simulink model "calcul_SA_SR"  (R2024b)
settings: Solver=VariableStepAuto  StartTime=0.0  StopTime=10.0  RelTol=1e-3
values from neighbouring files (symbols this model uses):
  Re = 0.47/2    (= 0.235)    [main_data_vehicle.m]
settings Model: Creator=marti  LastModifiedBy=marti

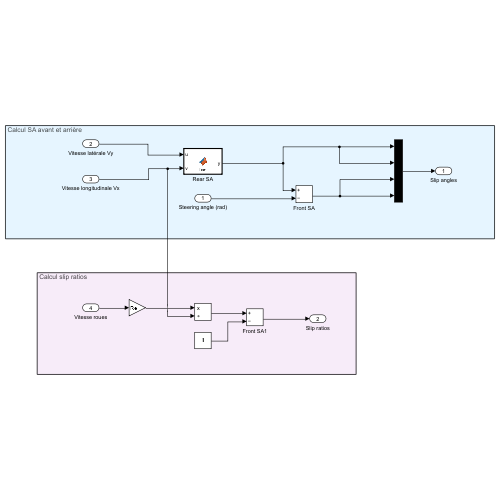
[thumbnail: Simulink's stored preview of the top-level diagram]
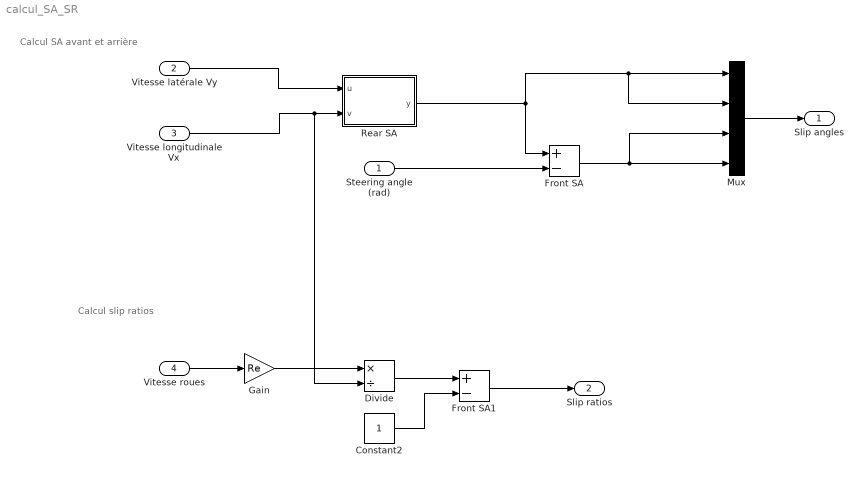
== system calcul_SA_SR ==
  note: Calcul slip ratios
  note: Calcul SA avant et arrière
  Steering angle (rad) : Inport
  Vitesse latérale Vy : Inport  Port=2
  Vitesse longitudinale Vx : Inport  Port=3
  Vitesse roues : Inport  Port=4
  Constant2 : Constant
  Divide : Product  Inputs=*/
  Front SA : Sum  Inputs=+-
  Front SA1 : Sum  Inputs=+-
  Gain : Gain  Gain=Re
  Mux : Mux
  Rear SA : MATLAB Function  TreatAsAtomicUnit=on
  Slip angles : Outport
  Slip ratios : Outport  Port=2
  wires:
  Vitesse latérale Vy/1 -> Rear SA/1(u)
  Steering angle (rad)/1 -> Front SA/2
  Rear SA/1(y) -> Front SA/1, Mux/2, Mux/1
  Front SA/1 -> Mux/3, Mux/4
  Mux/1 -> Slip angles/1
  Gain/1 -> Divide/1
  Divide/1 -> Front SA1/1
  Constant2/1 -> Front SA1/2
  Vitesse roues/1 -> Gain/1
  Vitesse longitudinale Vx/1 -> Divide/2, Rear SA/2(v)
  Front SA1/1 -> Slip ratios/1

== matlab function calcul_SA_SR/Rear SA ==
  data: u input; y output; v input
function y = fcn(u, v)

y = atan(u/v);
end
